simulink model "DiscreteControllerOnlyWithSFSaturation"  (Simulink 8.1)
settings: Solver=ode45  StartTime=0.0  StopTime=10.0  RelTol=1e-3
settings Model: Creator=root  LastModifiedBy=meta
settings DataIOCC: SignalLoggingSaveFormat=Dataset
settings OptimizationCC: ExpressionDepthLimit=128
settings DebuggingCC: FcnCallInpInsideContextMsg=EnableAllAsError
settings GRTTargetCC: CombineOutputUpdateFcns=on  GRTInterface=off

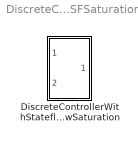
== system DiscreteControllerOnlyWithSFSaturation ==
  DiscreteControllerWithStateflowSaturation : Subsystem

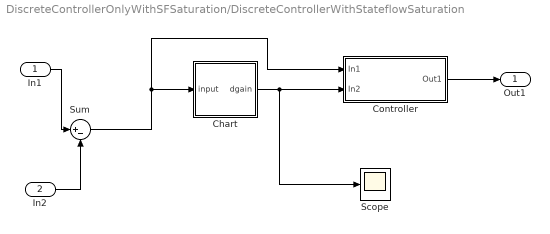
== system DiscreteControllerOnlyWithSFSaturation/DiscreteControllerWithStateflowSaturation ==
  In1 : Inport  OutDataTypeStr=double
  In2 : Inport  Port=2  OutDataTypeStr=double
  Chart : Stateflow chart  TreatAsAtomicUnit=on
  Controller : Subsystem
  Scope : Scope
      settings: SaveName=ScopeData2
  Sum : Sum  Inputs=|+-
  Out1 : Outport  OutDataTypeStr=double
  wires:
  Controller/1(Out1) -> Out1/1
  In1/1 -> Sum/1
  Chart/1(dgain) -> Scope/1, Controller/2(In2)
  Sum/1 -> Controller/1(In1), Chart/1(input)
  In2/1 -> Sum/2

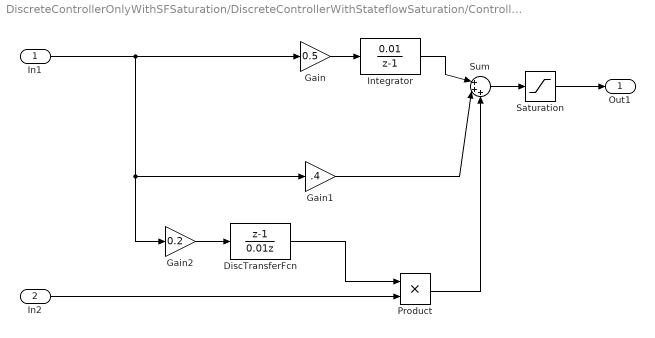
== system DiscreteControllerOnlyWithSFSaturation/DiscreteControllerWithStateflowSaturation/Controller ==
  In1 : Inport
  In2 : Inport  Port=2
  DiscTransferFcn : DiscreteTransferFcn  Numerator=[1 -1]  Denominator=[0.01 0]  SampleTime=0.01
  Gain : Gain  Gain=0.5
  Gain1 : Gain  Gain=.4
  Gain2 : Gain  Gain=0.2
  Integrator : DiscreteTransferFcn  Numerator=[0.01]  Denominator=[1 -1]  SampleTime=0.01
  Product : Product
  Saturation : Saturate  UpperLimit=10  LowerLimit=0
  Sum : Sum  Inputs=|+++
  Out1 : Outport
  wires:
  In1/1 -> Gain2/1, Gain1/1, Gain/1
  Gain/1 -> Integrator/1
  Integrator/1 -> Sum/1
  Gain1/1 -> Sum/2
  Sum/1 -> Saturation/1
  In2/1 -> Product/2
  Saturation/1 -> Out1/1
  Gain2/1 -> DiscTransferFcn/1
  DiscTransferFcn/1 -> Product/1
  Product/1 -> Sum/3

== stateflow chart DiscreteControllerWithStateflowSaturation/Chart ==
  state GainOn
    entry: dgain = 1
  state GainOff
    entry: dgain = 0
  (default) -> GainOn : {dgain = 1}
  GainOff -> GainOn : [input > 6]
  GainOn -> GainOff : [input < 2]
  data: input input double; dgain output double
